simulink model "DSB_AMVariableIndex"  (R2018a)
settings: Solver=VariableStepAuto  StartTime=0.0  StopTime=2  RelTol=1e-3
libraries: dsparch4 x1
settings Model: Creator=Neo  LastModifiedBy=Neo

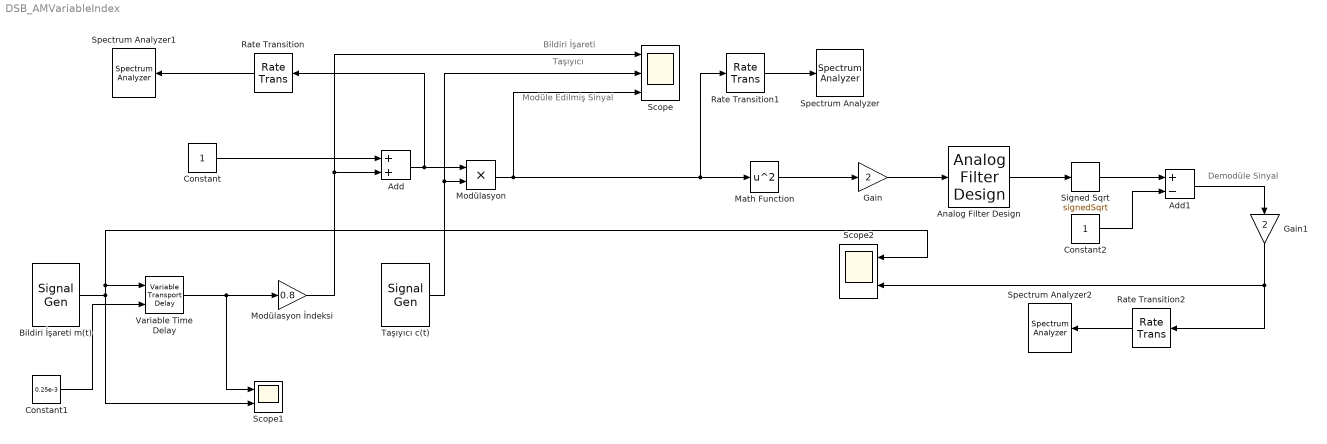
== system DSB_AMVariableIndex ==
  note: Demodüle Sinyal
  note: Modüle Edilmiş Sinyal
  note: Taşıyıcı
  note: Bildiri İşareti
  Add : Sum
  Add1 : Sum  Inputs=+-
  Analog Filter Design : dsparch4/Analog Filter Design  method=Butterworth  filttype=Lowpass  N=1  Wlo=2*pi*5000  Whi=80  Rp=2  Rs=40
  Bildiri İşareti m(t) : SignalGenerator  Frequency=1000
  Constant : Constant
  Constant1 : Constant  Value=0.25e-3
  Constant2 : Constant
  Gain : Gain  Gain=2
  "Gain1 " : Gain  Gain=2
  Math Function : Math  Operator=square  SaturateOnIntegerOverflow=on
  Modülasyon : Product
  Modülasyon İndeksi : Gain  Gain=0.8
  Rate Transition : RateTransition  OutPortSampleTime=0.00001
  Rate Transition1 : RateTransition  OutPortSampleTime=1/100000
  Rate Transition2 : RateTransition  OutPortSampleTime=1/100000
  Scope : Scope  NumInputPorts=3
  Scope1 : Scope  NumInputPorts=2
  Scope2 : Scope  NumInputPorts=2
  Signed Sqrt : Sqrt  Operator=signedSqrt  SaturateOnIntegerOverflow=on
  Spectrum Analyzer : SpectrumAnalyzer
  Spectrum Analyzer1 : SpectrumAnalyzer
  Spectrum Analyzer2 : SpectrumAnalyzer
  Taşıyıcı c(t) : SignalGenerator  Frequency=10000
  Variable Time Delay : VariableTransportDelay  MaximumDelay=10
  wires:
  Modülasyon İndeksi/1 -> Scope/1, Add/2
  Add/1 -> Rate Transition/1, Modülasyon/1
  Constant/1 -> Add/1
  Rate Transition1/1 -> Spectrum Analyzer/1
  Constant1/1 -> Variable Time Delay/2
  Variable Time Delay/1 -> Modülasyon İndeksi/1, Scope1/1
  Rate Transition/1 -> Spectrum Analyzer1/1
  Bildiri İşareti m(t)/1 -> Scope2/1, Variable Time Delay/1, Scope1/2
  Taşıyıcı c(t)/1 -> Modülasyon/2, Scope/2
  Math Function/1 -> Gain/1
  Gain/1 -> Analog Filter Design/1
  Analog Filter Design/1 -> Signed Sqrt/1
  Signed Sqrt/1 -> Add1/1
  Constant2/1 -> Add1/2
  Add1/1 -> "Gain1 "/1
  "Gain1 "/1 -> Scope2/2, Rate Transition2/1
  Rate Transition2/1 -> Spectrum Analyzer2/1
  Modülasyon/1 -> Rate Transition1/1, Math Function/1, Scope/3
